simulink subsystem "DCDCConverterSSC"  (R2024b)
settings: Solver=VariableStepAuto  StartTime=0.0  StopTime=10.0  RelTol=1e-3
undefined symbols (not defined in the file): BattNeg, BattPos, EnvAirTemp, HVDCNeg, HVDCPos, PlntBattNumCellSer, PlntBattOpenCirctVolt, PlntBattSocInit, PlntBattTempBpt, PlntBattTempInitDegC, PlntBattVoltSocBpt, PlntDCDCVoltInit
libraries: fl_lib x15, nesl_utility x2, ee_lib x1, nesl_utility_internal x1
settings Model: ModifiedByFormat=The MathWorks, Inc.  Creator=The MathWorks, Inc.  LastModifiedBy=The MathWorks, Inc.
settings OptimizationCC: ReuseModelBlockBuffer=off
settings DebuggingCC: SubsystemReferenceDiagnosticForUnitTest=warning
settings RTWCC: GPUComputeCapability=3.5

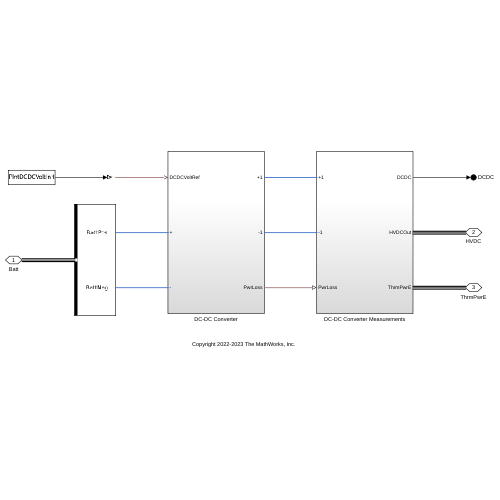
[thumbnail: Simulink's stored preview of the top-level diagram]
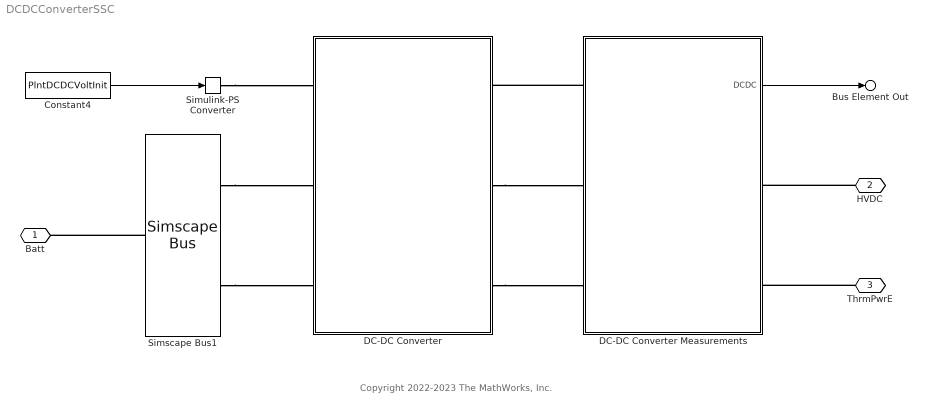
== system DCDCConverterSSC ==
  note: Copyright 2022-2023 The MathWorks, Inc.
  Constant4 : Constant  Value=PlntDCDCVoltInit  SampleTime=-1
  DC-DC Converter : Subsystem
  DC-DC Converter Measurements : Subsystem
  Simscape Bus1 : SimscapeBus  HierarchyStrings=BattPos;BattNeg
  Simulink-PS Converter : nesl_utility_internal/Simulink-PS Converter  PhysicalDomain=network_engine_domain  SubClassName=ps_input  LeftPortType=input  RightPortType=output  PseudoPeriodic=off  Frequencies=[]  NoiseDistribution=none  NoiseParameters=[]  Unit=1  AffineConversion=off  FilteringAndDerivatives=provide  SimscapeFilterOrder=1  InputFilterTimeConstant=0.001  UdotUserProvided=0
  Batt : PMIOPort  Side=Left
  HVDC : PMIOPort  Port=2  Side=Right
  ThrmPwrE : PMIOPort  Port=3  Side=Right
  Bus Element Out : Outport  PortName=DCDC
  wires:
  Constant4/1 -> Simulink-PS Converter/1
  DC-DC Converter Measurements/1(DCDC) -> Bus Element Out/1
  connections:
  Simulink-PS Converter/RConn1 -- DC-DC Converter/LConn1
  Simscape Bus1/LConn1 -- DC-DC Converter/LConn2
  Simscape Bus1/LConn2 -- DC-DC Converter/LConn3
  Simscape Bus1/RConn1 -- Batt/RConn1
  DC-DC Converter Measurements/LConn1 -- DC-DC Converter/RConn1
  ThrmPwrE/RConn1 -- DC-DC Converter Measurements/RConn2
  HVDC/RConn1 -- DC-DC Converter Measurements/RConn1
  DC-DC Converter/RConn2 -- DC-DC Converter Measurements/LConn2
  DC-DC Converter/RConn3 -- DC-DC Converter Measurements/LConn3

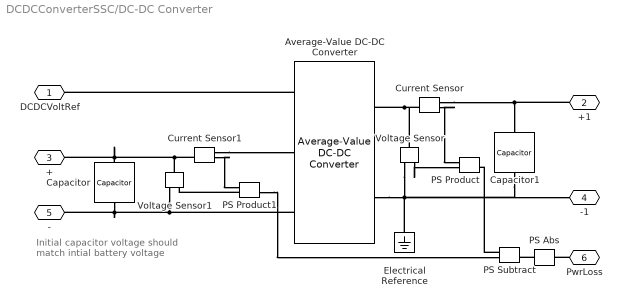
== system DCDCConverterSSC/DC-DC Converter ==
  note: Initial capacitor voltage
      | should match intial
      | battery voltage
  Average-Value DC-DC Converter : ee_lib/Semiconductors & Converters/Converters/Average-Value DC-DC Converter  control_option=ee.enum.converters.controlinput.voltage  converter_type=ee.enum.converters.dcdctype.buck  efficiency_option=ee.enum.converters.efficiency.constant  efficiency_fixed=PlntDCDCEff  i_vec=[0, 2, 5] A  efficiency_vec=[90, 95, 98]
      settings: InternalSimscapePortConfiguration="{\"Bottom\":[],\"Left\":[{\"id\":\"Vref\",\"label\":\"Vref\",\"type\":\"input\"},{\"id\":\"p1\",\"label\":\"1+\",\"type\":\"foundation.electrical.electrical\"},{\"id\":\"n1\",\"label\":\"1-\",\"type\":\"foundation.electrical.electrical\"}],\"Right\":[{\"id\":\"p2\",\"label\":\"2+\",\"type\":\"foundation.electrical.electrical\"},{\"id\":\"n2\",\"label\":\"2-\",\"type\":\"foundation.electrical.electrical\"}],\"Top\":[]}"
  Capacitor : fl_lib/Electrical/Electrical Elements/Capacitor  c=PlntDCDCFltrCap uF  r=PlntDCDCFltrRes Ohm  g=0 1/Ohm  i_specify=off  i_priority=None  i=0 A  i_nominal_specify=off  i_nominal_value=1  i_nominal_unit=A  v_specify=off  v_priority=None  v=0 V  v_nominal_specify=off  v_nominal_value=1  v_nominal_unit=V  vc_specify=on  vc_priority=High  vc=interp2(PlntBattTempBpt,PlntBattVoltSocBpt,PlntBattOpenCirctVolt*PlntBattNumCellSer,PlntBattTempInitDegC,PlntBattSocInit) V  vc_nominal_specify=off  vc_nominal_value=1  vc_nominal_unit=V
  Capacitor1 : fl_lib/Electrical/Electrical Elements/Capacitor  c=PlntDCDCFltrCap uF  r=PlntDCDCFltrRes Ohm  g=0 1/Ohm  i_specify=off  i_priority=None  i=0 A  i_nominal_specify=off  i_nominal_value=1  i_nominal_unit=A  v_specify=off  v_priority=None  v=0 V  v_nominal_specify=off  v_nominal_value=1  v_nominal_unit=V  vc_specify=on  vc_priority=High  vc=PlntDCDCVoltInit V  vc_nominal_specify=off  vc_nominal_value=1  vc_nominal_unit=V
  Current Sensor : fl_lib/Electrical/Electrical Sensors/Current Sensor
  Current Sensor1 : fl_lib/Electrical/Electrical Sensors/Current Sensor
  Electrical Reference : fl_lib/Electrical/Electrical Elements/Electrical Reference
  PS Abs : fl_lib/Physical Signals/Nonlinear Operators/PS Abs
      settings: InternalSimscapePortConfiguration="{\"Bottom\":[],\"Left\":[{\"id\":\"I\",\"label\":\"\",\"type\":\"input\"}],\"Right\":[{\"id\":\"O\",\"label\":\"\",\"type\":\"output\"}],\"Top\":[]}"
  PS Product : fl_lib/Physical Signals/Functions/PS Product
  PS Product1 : fl_lib/Physical Signals/Functions/PS Product
  PS Subtract : fl_lib/Physical Signals/Functions/PS Subtract
  Voltage Sensor : fl_lib/Electrical/Electrical Sensors/Voltage Sensor
  Voltage Sensor1 : fl_lib/Electrical/Electrical Sensors/Voltage Sensor
  DCDCVoltRef : PMIOPort  Side=Left
  +1 : PMIOPort  Port=2  Side=Right
  + : PMIOPort  Port=3  Side=Left
  -1 : PMIOPort  Port=4  Side=Right
  - : PMIOPort  Port=5  Side=Left
  PwrLoss : PMIOPort  Port=6  Side=Right
  connections:
  PS Product1/LConn2 -- Voltage Sensor1/RConn1
  Current Sensor1/RConn1 -- PS Product1/LConn1
  Current Sensor1/RConn2 -- Average-Value DC-DC Converter/LConn2
  Voltage Sensor/RConn1 -- PS Product/LConn2
  Current Sensor/RConn1 -- PS Product/LConn1
  Voltage Sensor/LConn1 -- Current Sensor/LConn1 -- Average-Value DC-DC Converter/RConn1
  Voltage Sensor1/RConn2 -- -/RConn1 -- Capacitor/RConn1 -- Average-Value DC-DC Converter/LConn3
  Current Sensor1/LConn1 -- Voltage Sensor1/LConn1 -- +/RConn1 -- Capacitor/LConn1
  Average-Value DC-DC Converter/LConn1 -- DCDCVoltRef/RConn1
  Voltage Sensor/RConn2 -- Capacitor1/RConn1 -- -1/RConn1 -- Electrical Reference/LConn1 -- Average-Value DC-DC Converter/RConn2
  Current Sensor/RConn2 -- Capacitor1/LConn1 -- +1/RConn1
  PS Subtract/LConn1 -- PS Product/RConn1
  PS Product1/RConn1 -- PS Subtract/LConn2
  PS Abs/LConn1 -- PS Subtract/RConn1
  PwrLoss/RConn1 -- PS Abs/RConn1

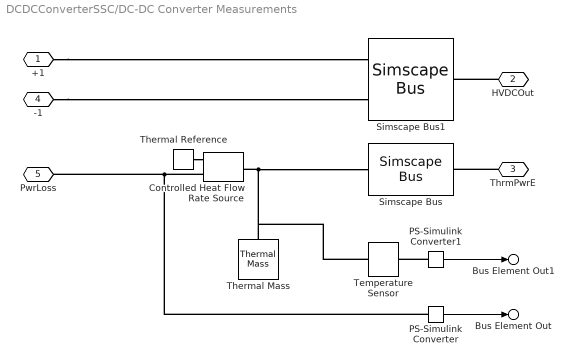
== system DCDCConverterSSC/DC-DC Converter Measurements ==
  Controlled Heat Flow Rate Source : fl_lib/Thermal/Thermal Sources/Controlled Heat Flow Rate Source
  PS-Simulink Converter : nesl_utility/PS-Simulink Converter  PhysicalDomain=network_engine_domain  SubClassName=ps_output  LeftPortType=input  RightPortType=output  PseudoPeriodic=off  Frequencies=[]  VectorFormat=inherit  Unit=inherit  AffineConversion=off
  PS-Simulink Converter1 : nesl_utility/PS-Simulink Converter  PhysicalDomain=network_engine_domain  SubClassName=ps_output  LeftPortType=input  RightPortType=output  PseudoPeriodic=off  Frequencies=[]  VectorFormat=inherit  Unit=inherit  AffineConversion=off
  Simscape Bus : SimscapeBus  HierarchyStrings=ThrmPwrE1
  Simscape Bus1 : SimscapeBus  HierarchyStrings=HVDCPos;HVDCNeg
  Temperature Sensor : fl_lib/Thermal/Thermal Sensors/Temperature Sensor  temperature_measure=foundation.enum.MeasurementReference.absolute
      settings: InternalSimscapePortConfiguration="{\"Bottom\":[],\"Left\":[{\"id\":\"A\",\"label\":\"A\",\"type\":\"foundation.thermal.thermal\"}],\"Right\":[{\"id\":\"T\",\"label\":\"T\",\"type\":\"output\"}],\"Top\":[]}"
  Thermal Mass : fl_lib/Thermal/Thermal Elements/Thermal Mass  mass_type=foundation.enum.constant_variable.constant  mass=PlntDCDCMass kg  sp_heat=PlntEMCp J/(K*kg)  mass_min=1e-6 kg  num_ports=foundation.enum.numPorts2.one  m_specify=off  m_priority=High  m=1 kg  m_nominal_specify=off  m_nominal_value=1  m_nominal_unit=kg  T_specify=on  T_priority=High  T=EnvAirTemp K  T_nominal_specify=off  T_nominal_value=1  T_nominal_unit=K  Q_specify=off  Q_priority=None  Q=0 W  Q_nominal_specify=off  Q_nominal_value=1  Q_nominal_unit=W
  Thermal Reference : fl_lib/Thermal/Thermal Elements/Thermal Reference
  +1 : PMIOPort  Side=Left
  HVDCOut : PMIOPort  Port=2  Side=Right
  ThrmPwrE : PMIOPort  Port=3  Side=Right
  -1 : PMIOPort  Port=4  Side=Left
  PwrLoss : PMIOPort  Port=5  Side=Left
  Bus Element Out : Outport  PortName=DCDC  Element=PwrELoss
  Bus Element Out1 : Outport  PortName=DCDC  Element=PwrETemp
  wires:
  PS-Simulink Converter1/1 -> Bus Element Out1/1
  PS-Simulink Converter/1 -> Bus Element Out/1
  connections:
  +1/RConn1 -- Simscape Bus1/LConn1
  HVDCOut/RConn1 -- Simscape Bus1/RConn1
  Thermal Reference/LConn1 -- Controlled Heat Flow Rate Source/RConn2
  -1/RConn1 -- Simscape Bus1/LConn2
  Controlled Heat Flow Rate Source/LConn1 -- Simscape Bus/LConn1 -- Temperature Sensor/LConn1 -- Thermal Mass/LConn1
  ThrmPwrE/RConn1 -- Simscape Bus/RConn1
  PS-Simulink Converter1/LConn1 -- Temperature Sensor/RConn1
  Controlled Heat Flow Rate Source/RConn1 -- PwrLoss/RConn1 -- PS-Simulink Converter/LConn1
